simulink model "Ex_4_Alcancar_sim"  (R2024b)
settings: Solver=VariableStepAuto  StartTime=0.0  StopTime=10.0  RelTol=1e-3
values from neighbouring files (symbols this model uses):
  xg = [6 9 pi]    [Ex4_alcancar.m]    (also in Ex4_test.m)
libraries: roblocks x1, simulink x1
settings Model: Creator=barba  LastModifiedBy=caugu

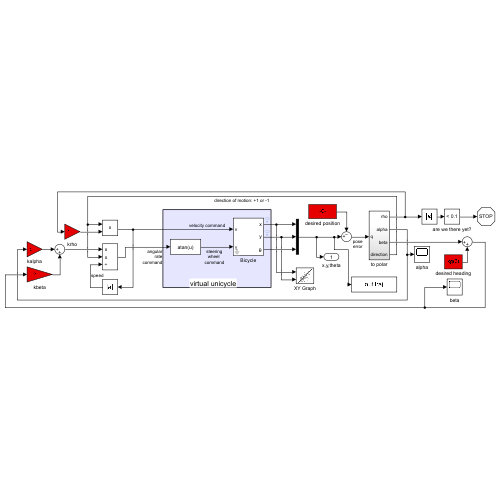
[thumbnail: Simulink's stored preview of the top-level diagram]
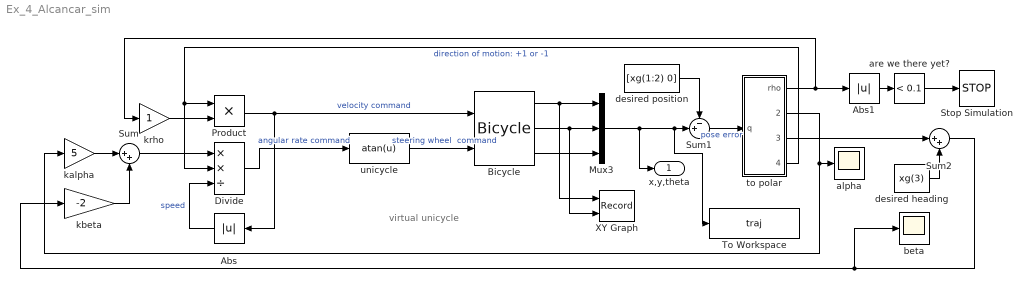
== system Ex_4_Alcancar_sim ==
  note: virtual unicycle
  Abs : Abs  SaturateOnIntegerOverflow=off
  Abs1 : Abs  SaturateOnIntegerOverflow=off
  Bicycle : roblocks/Vehicles/Bicycle  vlim=1  accel=1  alim=1  steer_rate=Inf  L=1  x0=x0
  Divide : Product  Inputs=**/
  Mux3 : Mux  Inputs=3
  Product : Product  RndMeth=Zero
  Stop Simulation : Stop
  Sum : Sum  Inputs=|++
  Sum1 : Sum  Inputs=-+|
  Sum2 : Sum  Inputs=|++
  To Workspace : ToWorkspace  VariableName=traj  SampleTime=-1
  XY Graph : Record  FileSettingsInternal="{\"entries\":[{\"content\":{\"excelSettings\":{\"content\":{},\"type\":\"Streamout.ExcelSettings\"}},\"type\":\"Streamout.FileSettingStorage\",\"uuid\":\"\"}],\"packageUris\":[\"http:\\/\\/schema.mathworks.com\\/mf0\\/streamout_blocks\\/R2020a\"],\"version\":\"1.0\"}"  Layout=[1 1]  SignalsInternal="{\"entries\":[{\"content\":{\"signals\":[{\"content\":{\"blockPath\":[],\"dimensions\":[1],\"domain\":\"\",\"lineColor\":\"#a2142f\",\"lineWidth\":2,\"port\":1,\"sid\":[\"\"],\"signalID\":1,\"signalName\":\"Bicycle:1\"},\"type\":\"RecordBlkView.Signal\",\"uuid\":\"\"},{\"content\":{\"blockPath\":[],\"dimensions\":[1],\"domain\":\"\",\"lineColor\":\"#139fff\",\"lineWidth\":2,\"port\":2,\"sid\":[\"\"],\"signalID\":2,\"signalName\":\"Bicycle:2\"},\"type\":\"RecordBlkView.Signal\",\"uuid\":\"\"}]},\"type\":\"RecordBlkView.InputSignals\",\"uuid\":\"\"}],\"packageUris\":[\"http:\\/\\/schema.mathworks.com\\/mf0\\/streamout_blocks\\/R2020a\"],\"version\":\"1.0\"}"  VisualizationBindings="{\"xyplotplugin\":{\"info\":[{\"series\":[{\"bindingParametersList\":[{\"parameter\":\"X-Axis\",\"signalID\":4159,\"signalName\":\"Bicycle:1\"},{\"parameter\":\"Y-Axis\",\"signalID\":4163,\"signalName\":\"Bicycle:2\"}],\"seriesID\":0}],\"subplotID\":1}]}}"  CompatibilityTag=XY
  alpha : Scope
  are we there yet? : simulink/Logic and Bit Operations/Compare To Constant  relop=<  const=0.1  OutDataTypeStr=boolean
  beta : Scope
  desired heading : Constant  Value=xg(3)
  desired position : Constant  Value=[xg(1:2) 0]
  kalpha : Gain  Gain=5
  kbeta : Gain  Gain=-2
  krho : Gain
  to polar : Subsystem
  "unicycle " : Fcn  Expr=atan(u)
  x,y,theta : Outport  VectorParamsAs1DForOutWhenUnconnected=off
  wires:
  to polar/3(beta) -> Sum2/1
  "unicycle "/1 -> Bicycle/2  "steering wheel  command"
  Bicycle/3 -> Mux3/3
  Mux3/1 -> x,y,theta/1, To Workspace/1, Sum1/2
  to polar/1(rho) -> Abs1/1, krho/1
  Abs/1 -> Divide/3  "speed"
  Product/1 -> Bicycle/1, Abs/1  "velocity command"
  krho/1 -> Product/2
  Sum/1 -> Divide/1
  Divide/1 -> "unicycle "/1  "angular rate command"
  to polar/2(alpha) -> kalpha/1, alpha/1
  Bicycle/2 -> XY Graph/2, Mux3/2
  Bicycle/1 -> XY Graph/1, Mux3/1
  Abs1/1 -> are we there yet?/1
  are we there yet?/1 -> Stop Simulation/1
  desired position/1 -> Sum1/1
  Sum2/1 -> kbeta/1, beta/1
  desired heading/1 -> Sum2/2
  to polar/4(direction) -> Product/1, Divide/2  "direction of motion: +1 or -1"
  kalpha/1 -> Sum/1
  kbeta/1 -> Sum/2
  Sum1/1 -> to polar/1(q)  "pose error"

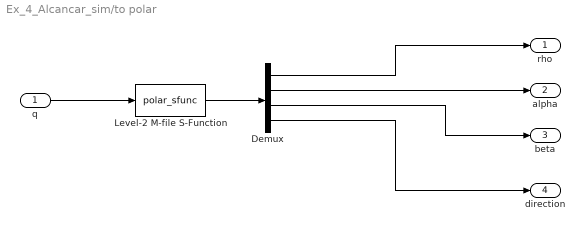
== system Ex_4_Alcancar_sim/to polar ==
  q : Inport
  Demux : Demux
  Level-2 M-file S-Function : M-S-Function  FunctionName=polar_sfunc
  rho : Outport  VectorParamsAs1DForOutWhenUnconnected=off
  alpha : Outport  Port=2  VectorParamsAs1DForOutWhenUnconnected=off
  beta : Outport  Port=3  VectorParamsAs1DForOutWhenUnconnected=off
  direction : Outport  Port=4  VectorParamsAs1DForOutWhenUnconnected=off
  wires:
  Demux/3 -> beta/1
  q/1 -> Level-2 M-file S-Function/1
  Level-2 M-file S-Function/1 -> Demux/1
  Demux/1 -> rho/1
  Demux/2 -> alpha/1
  Demux/4 -> direction/1
